simulink model "Multi_agent_system"  (R2016b)
settings: Solver=VariableStepAuto  StartTime=0.0  StopTime=10  RelTol=1e-3
undefined symbols (not defined in the file or in its folder): A, Kr, Kv, n, r, v_initial, x_initial
settings Model: Creator=kvlton  LastModifiedBy=kvlton

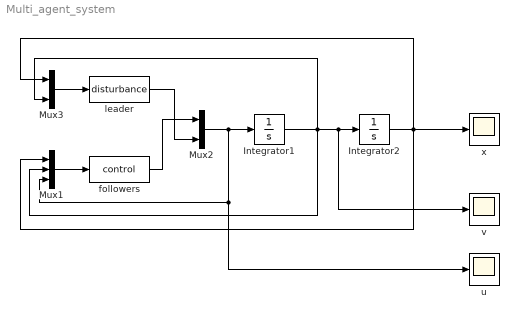
== system Multi_agent_system ==
  Integrator1 : Integrator  InitialCondition=v_initial
  Integrator2 : Integrator  InitialCondition=x_initial
  Mux1 : Mux  Inputs=3
  Mux2 : Mux  Inputs=2
  Mux3 : Mux  Inputs=2
  followers : S-Function  FunctionName=control  Parameters=A,n,r,Kr,Kv  SFunctionDeploymentMode=off  EnableBusSupport=off
  leader : S-Function  FunctionName=disturbance  Parameters=n  SFunctionDeploymentMode=off  EnableBusSupport=off
  u : Scope
  v : Scope
  x : Scope
  wires:
  Mux1/1 -> followers/1
  Integrator2/1 -> Mux3/1, x/1, Mux1/1
  Mux2/1 -> Integrator1/1, Mux1/3, u/1
  Mux3/1 -> leader/1
  Integrator1/1 -> Mux3/2, v/1, Integrator2/1, Mux1/2
  leader/1 -> Mux2/2
  followers/1 -> Mux2/1
